simulink subsystem "SegmentSOC"  (R2021a)
settings: Solver=VariableStepAuto  StartTime=0.0  StopTime=10.0  RelTol=1e-3
settings Model: Creator=mirko  LastModifiedBy=mirko

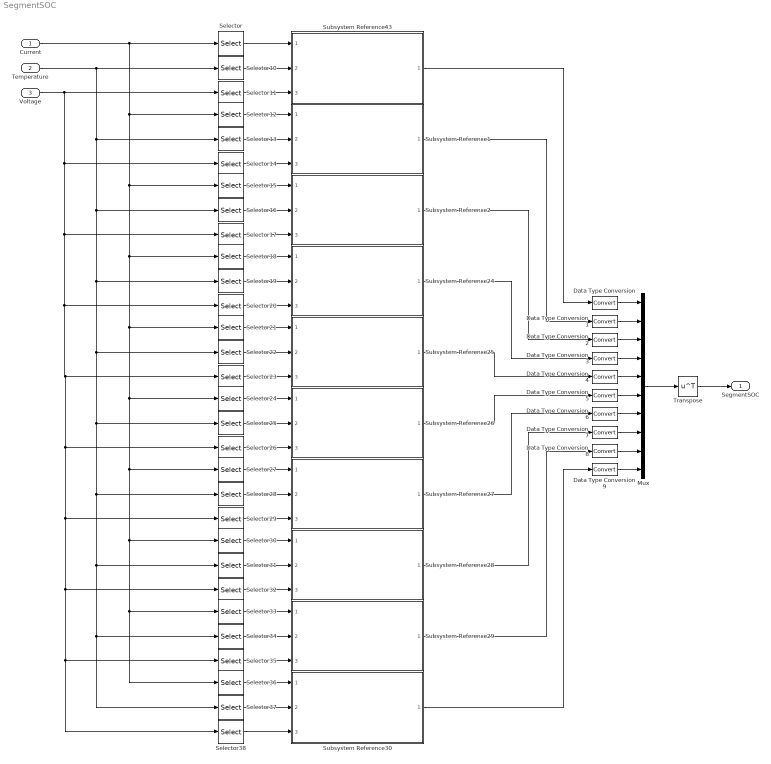
== system SegmentSOC ==
  Current : Inport
  Temperature : Inport  Port=2
  Voltage : Inport  Port=3
  Data Type Conversion{,1..9} (10 alike) : DataTypeConversion
  Mux : Mux  Inputs=10
  Selector : Selector  InputPortWidth=10  IndexOptions=Index vector (dialog)  Indices=1  OutputSizes=1
  Selector10 : Selector  InputPortWidth=10  IndexOptions=Index vector (dialog)  Indices=1  OutputSizes=1
  Selector11 : Selector  InputPortWidth=10  IndexOptions=Index vector (dialog)  Indices=1  OutputSizes=1
  Selector12 : Selector  InputPortWidth=10  IndexOptions=Index vector (dialog)  Indices=2  OutputSizes=1
  Selector13 : Selector  InputPortWidth=10  IndexOptions=Index vector (dialog)  Indices=2  OutputSizes=1
  Selector14 : Selector  InputPortWidth=10  IndexOptions=Index vector (dialog)  Indices=2  OutputSizes=1
  Selector15 : Selector  InputPortWidth=10  IndexOptions=Index vector (dialog)  Indices=3  OutputSizes=1
  Selector16 : Selector  InputPortWidth=10  IndexOptions=Index vector (dialog)  Indices=3  OutputSizes=1
  Selector17 : Selector  InputPortWidth=10  IndexOptions=Index vector (dialog)  Indices=3  OutputSizes=1
  Selector18 : Selector  InputPortWidth=10  IndexOptions=Index vector (dialog)  Indices=4  OutputSizes=1
  Selector19 : Selector  InputPortWidth=10  IndexOptions=Index vector (dialog)  Indices=4  OutputSizes=1
  Selector20 : Selector  InputPortWidth=10  IndexOptions=Index vector (dialog)  Indices=4  OutputSizes=1
  Selector21 : Selector  InputPortWidth=10  IndexOptions=Index vector (dialog)  Indices=5  OutputSizes=1
  Selector22 : Selector  InputPortWidth=10  IndexOptions=Index vector (dialog)  Indices=5  OutputSizes=1
  Selector23 : Selector  InputPortWidth=10  IndexOptions=Index vector (dialog)  Indices=5  OutputSizes=1
  Selector24 : Selector  InputPortWidth=10  IndexOptions=Index vector (dialog)  Indices=6  OutputSizes=1
  Selector25 : Selector  InputPortWidth=10  IndexOptions=Index vector (dialog)  Indices=6  OutputSizes=1
  Selector26 : Selector  InputPortWidth=10  IndexOptions=Index vector (dialog)  Indices=6  OutputSizes=1
  Selector27 : Selector  InputPortWidth=10  IndexOptions=Index vector (dialog)  Indices=7  OutputSizes=1
  Selector28 : Selector  InputPortWidth=10  IndexOptions=Index vector (dialog)  Indices=7  OutputSizes=1
  Selector29 : Selector  InputPortWidth=10  IndexOptions=Index vector (dialog)  Indices=7  OutputSizes=1
  Selector30 : Selector  InputPortWidth=10  IndexOptions=Index vector (dialog)  Indices=8  OutputSizes=1
  Selector31 : Selector  InputPortWidth=10  IndexOptions=Index vector (dialog)  Indices=8  OutputSizes=1
  Selector32 : Selector  InputPortWidth=10  IndexOptions=Index vector (dialog)  Indices=8  OutputSizes=1
  Selector33 : Selector  InputPortWidth=10  IndexOptions=Index vector (dialog)  Indices=9  OutputSizes=1
  Selector34 : Selector  InputPortWidth=10  IndexOptions=Index vector (dialog)  Indices=9  OutputSizes=1
  Selector35 : Selector  InputPortWidth=10  IndexOptions=Index vector (dialog)  Indices=9  OutputSizes=1
  Selector36 : Selector  InputPortWidth=10  IndexOptions=Index vector (dialog)  Indices=10  OutputSizes=1
  Selector37 : Selector  InputPortWidth=10  IndexOptions=Index vector (dialog)  Indices=10  OutputSizes=1
  Selector38 : Selector  InputPortWidth=10  IndexOptions=Index vector (dialog)  Indices=10  OutputSizes=1
  Subsystem Reference{1..2,24..30,43} (10 alike) : Subsystem  ReferencedSubsystem=Single_Cell_SOC_Estimation
  Transpose : Math  Operator=transpose  SaturateOnIntegerOverflow=on
  "SegmentSOC " : Outport
  wires:
  Transpose/1 -> "SegmentSOC "/1
  Subsystem Reference26/1 -> Data Type Conversion5/1
  Selector34/1 -> Subsystem Reference29/2
  Voltage/1 -> Selector11/1, Selector14/1, Selector17/1, Selector20/1, Selector23/1, Selector26/1, Selector29/1, Selector32/1, Selector38/1, Selector35/1
  Current/1 -> Selector/1, Selector12/1, Selector18/1, Selector24/1, Selector27/1, Selector30/1, Selector33/1, Selector36/1, Selector21/1, Selector15/1
  Selector13/1 -> Subsystem Reference1/2
  Subsystem Reference1/1 -> Data Type Conversion1/1
  Subsystem Reference2/1 -> Data Type Conversion2/1
  Selector36/1 -> Subsystem Reference30/1
  Temperature/1 -> Selector10/1, Selector13/1, Selector16/1, Selector19/1, Selector22/1, Selector25/1, Selector28/1, Selector31/1, Selector34/1, Selector37/1
  Selector19/1 -> Subsystem Reference24/2
  Selector11/1 -> Subsystem Reference43/3
  Selector29/1 -> Subsystem Reference27/3
  Subsystem Reference27/1 -> Data Type Conversion6/1
  Subsystem Reference25/1 -> Data Type Conversion4/1
  Selector15/1 -> Subsystem Reference2/1
  Selector18/1 -> Subsystem Reference24/1
  Subsystem Reference28/1 -> Data Type Conversion7/1
  Selector27/1 -> Subsystem Reference27/1
  Selector20/1 -> Subsystem Reference24/3
  Subsystem Reference30/1 -> Data Type Conversion9/1
  Selector21/1 -> Subsystem Reference25/1
  Subsystem Reference43/1 -> Data Type Conversion/1
  Mux/1 -> Transpose/1
  Subsystem Reference29/1 -> Data Type Conversion8/1
  Subsystem Reference24/1 -> Data Type Conversion3/1
  Selector10/1 -> Subsystem Reference43/2
  Selector17/1 -> Subsystem Reference2/3
  Selector28/1 -> Subsystem Reference27/2
  Selector/1 -> Subsystem Reference43/1
  Selector32/1 -> Subsystem Reference28/3
  Selector35/1 -> Subsystem Reference29/3
  Selector37/1 -> Subsystem Reference30/2
  Selector31/1 -> Subsystem Reference28/2
  Selector16/1 -> Subsystem Reference2/2
  Selector33/1 -> Subsystem Reference29/1
  Selector22/1 -> Subsystem Reference25/2
  Selector23/1 -> Subsystem Reference25/3
  Selector25/1 -> Subsystem Reference26/2
  Selector26/1 -> Subsystem Reference26/3
  Selector24/1 -> Subsystem Reference26/1
  Selector30/1 -> Subsystem Reference28/1
  Selector14/1 -> Subsystem Reference1/3
  Selector38/1 -> Subsystem Reference30/3
  Selector12/1 -> Subsystem Reference1/1
  Data Type Conversion/1 -> Mux/1
  Data Type Conversion2/1 -> Mux/3
  Data Type Conversion1/1 -> Mux/2
  Data Type Conversion3/1 -> Mux/4
  Data Type Conversion4/1 -> Mux/5
  Data Type Conversion5/1 -> Mux/6
  Data Type Conversion6/1 -> Mux/7
  Data Type Conversion7/1 -> Mux/8
  Data Type Conversion8/1 -> Mux/9
  Data Type Conversion9/1 -> Mux/10
